simulink model "firebreak_microgrid"  (R2026a)
settings: Solver=ode45  StopTime=86400  MaxStep=0.1
settings Model: Creator=bawan  LastModifiedBy=bawan

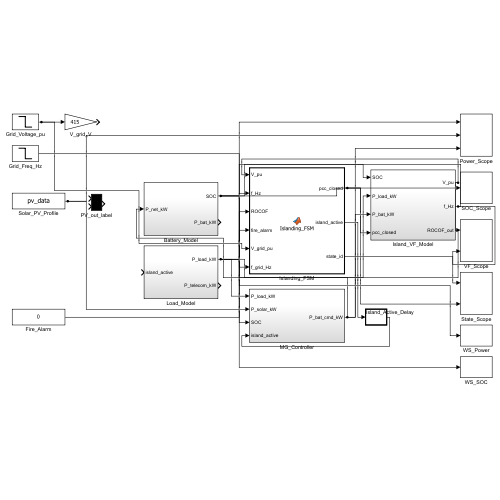
[thumbnail: Simulink's stored preview of the top-level diagram]
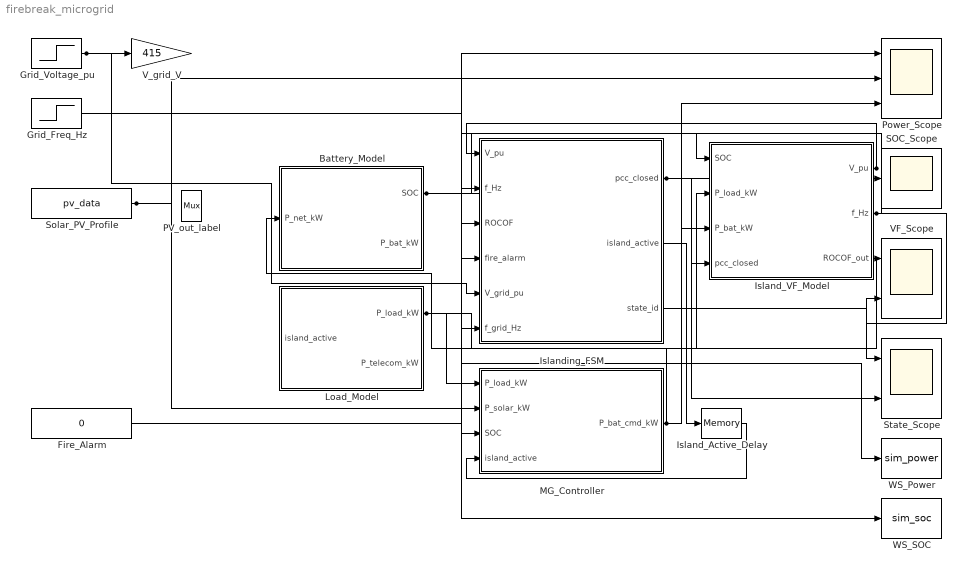
== system firebreak_microgrid ==
  Battery_Model : Subsystem
  Fire_Alarm : Constant  Value=0
  Grid_Freq_Hz : Step  Time=61200  InitialValue=50  FinalValue=0  SampleTime=0
  Grid_Voltage_pu : Step  Time=61200  InitialValue=1.0  FinalValue=0.0  SampleTime=0
  Island_Active_Delay : Memory
  Island_VF_Model : Subsystem
  Islanding_FSM : MATLAB Function  TreatAsAtomicUnit=on
  Load_Model : Subsystem
  MG_Controller : Subsystem
  PV_out_label : Mux  Inputs=2
  Power_Scope : Scope  NumInputPorts=3
  SOC_Scope : Scope
  Solar_PV_Profile : FromWorkspace  VariableName=pv_data  OutputAfterFinalValue=Holding final value
  State_Scope : Scope  NumInputPorts=2
  VF_Scope : Scope  NumInputPorts=2
  V_grid_V : Gain  Gain=415
  WS_Power : ToWorkspace  VariableName=sim_power  SaveFormat=Timeseries  SampleTime=-1
  WS_SOC : ToWorkspace  VariableName=sim_soc  SaveFormat=Timeseries  SampleTime=-1
  wires:
  Grid_Voltage_pu/1 -> V_grid_V/1, Islanding_FSM/5(V_grid_pu)
  Solar_PV_Profile/1 -> MG_Controller/2(P_solar_kW), Power_Scope/2
  Load_Model/1(P_load_kW) -> MG_Controller/1(P_load_kW), Island_VF_Model/2(P_load_kW), Power_Scope/1, WS_Power/1
  Battery_Model/1(SOC) -> MG_Controller/3(SOC), Island_VF_Model/1(SOC), SOC_Scope/1, WS_SOC/1
  Islanding_FSM/2(island_active) -> Island_Active_Delay/1
  Island_Active_Delay/1 -> MG_Controller/4(island_active)
  MG_Controller/1(P_bat_cmd_kW) -> Island_VF_Model/3(P_bat_kW), Battery_Model/1(P_net_kW), Power_Scope/3
  Islanding_FSM/1(pcc_closed) -> Island_VF_Model/4(pcc_closed), State_Scope/2
  Fire_Alarm/1 -> Islanding_FSM/4(fire_alarm)
  Grid_Freq_Hz/1 -> Islanding_FSM/6(f_grid_Hz)
  Island_VF_Model/1(V_pu) -> Islanding_FSM/1(V_pu), VF_Scope/1
  Island_VF_Model/2(f_Hz) -> Islanding_FSM/2(f_Hz), VF_Scope/2
  Island_VF_Model/3(ROCOF_out) -> Islanding_FSM/3(ROCOF)
  Islanding_FSM/3(state_id) -> State_Scope/1

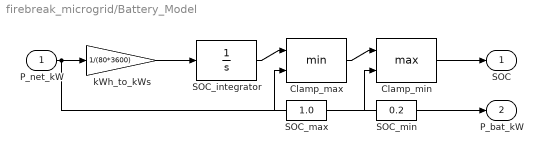
== system firebreak_microgrid/Battery_Model ==
  P_net_kW : Inport
  Clamp_max : MinMax  Inputs=2
  Clamp_min : MinMax  Function=max  Inputs=2
  SOC_integrator : Integrator  InitialCondition=1
  SOC_max : Constant  Value=1.0
  SOC_min : Constant  Value=0.2
  kWh_to_kWs : Gain  Gain=1/(80*3600)
  SOC : Outport
  P_bat_kW : Outport  Port=2
  wires:
  P_net_kW/1 -> kWh_to_kWs/1, P_bat_kW/1
  kWh_to_kWs/1 -> SOC_integrator/1
  SOC_integrator/1 -> Clamp_max/1
  SOC_max/1 -> Clamp_max/2
  Clamp_max/1 -> Clamp_min/1
  SOC_min/1 -> Clamp_min/2
  Clamp_min/1 -> SOC/1

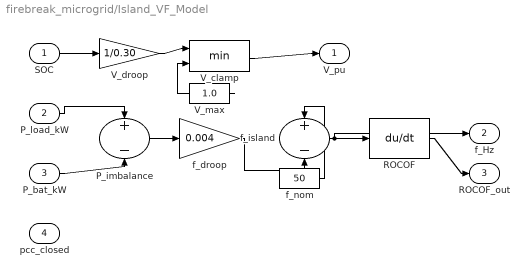
== system firebreak_microgrid/Island_VF_Model ==
  SOC : Inport
  P_load_kW : Inport  Port=2
  P_bat_kW : Inport  Port=3
  pcc_closed : Inport  Port=4
  P_imbalance : Sum  Inputs=+-
  ROCOF : Derivative
  V_clamp : MinMax  Inputs=2
  V_droop : Gain  Gain=1/0.30
  V_max : Constant  Value=1.0
  f_droop : Gain  Gain=0.004
  f_island : Sum  Inputs=+-
  f_nom : Constant  Value=50
  V_pu : Outport
  f_Hz : Outport  Port=2
  ROCOF_out : Outport  Port=3
  wires:
  SOC/1 -> V_droop/1
  V_droop/1 -> V_clamp/1
  V_max/1 -> V_clamp/2
  P_load_kW/1 -> P_imbalance/1
  P_bat_kW/1 -> P_imbalance/2
  P_imbalance/1 -> f_droop/1
  f_nom/1 -> f_island/1
  f_droop/1 -> f_island/2
  f_island/1 -> ROCOF/1, f_Hz/1
  V_clamp/1 -> V_pu/1
  ROCOF/1 -> ROCOF_out/1

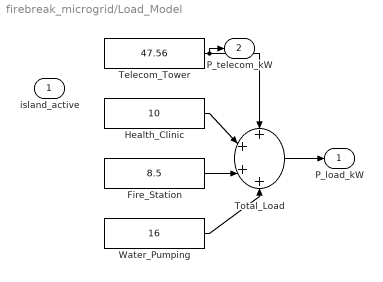
== system firebreak_microgrid/Load_Model ==
  island_active : Inport
  Fire_Station : Constant  Value=8.5
  Health_Clinic : Constant  Value=10
  Telecom_Tower : Constant  Value=47.56
  Total_Load : Sum  Inputs=++++
  Water_Pumping : Constant  Value=16
  P_load_kW : Outport
  P_telecom_kW : Outport  Port=2
  wires:
  Telecom_Tower/1 -> Total_Load/1, P_telecom_kW/1
  Health_Clinic/1 -> Total_Load/2
  Fire_Station/1 -> Total_Load/3
  Water_Pumping/1 -> Total_Load/4
  Total_Load/1 -> P_load_kW/1

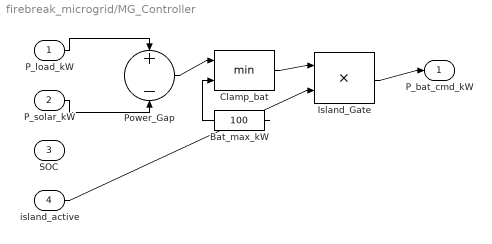
== system firebreak_microgrid/MG_Controller ==
  P_load_kW : Inport
  P_solar_kW : Inport  Port=2
  SOC : Inport  Port=3
  island_active : Inport  Port=4
  Bat_max_kW : Constant  Value=100
  Clamp_bat : MinMax  Inputs=2
  Island_Gate : Product
  Power_Gap : Sum  Inputs=+-
  P_bat_cmd_kW : Outport
  wires:
  P_load_kW/1 -> Power_Gap/1
  P_solar_kW/1 -> Power_Gap/2
  Power_Gap/1 -> Clamp_bat/1
  Bat_max_kW/1 -> Clamp_bat/2
  Clamp_bat/1 -> Island_Gate/1
  island_active/1 -> Island_Gate/2
  Island_Gate/1 -> P_bat_cmd_kW/1

== matlab function firebreak_microgrid/Islanding_FSM ==
  data: V_pu input; pcc_closed output; f_Hz input; ROCOF input; fire_alarm input; V_grid_pu input; f_grid_Hz input; island_active output; state_id output
function [pcc_closed, island_active, state_id] = Islanding_FSM(...
    V_pu, f_Hz, ROCOF, fire_alarm, V_grid_pu, f_grid_Hz)
%#codegen
% Islanding state machine for Firebreak Microgrid
% AS/NZS 4777.2 compliant loss-of-supply detection
%
% States:
%   0 = GRID_CONNECTED  — normal, PCC closed
%   1 = ISLANDED        — PCC open, battery supplies load
%   2 = RESYNC_CHECK    — grid back, checking conditions
%   3 = RECONNECTED     — PCC reclosed, back to grid

% Thresholds (AS/NZS 4777.2)
UV_thresh   = 0.85;   % Under-voltage (pu)
OV_thresh   = 1.10;   % Over-voltage (pu)
UF_thresh   = 49.0;   % Under-frequency (Hz)
OF_thresh   = 51.0;   % Over-frequency (Hz)
ROCOF_thresh= 1.0;    % Rate of change of frequency (Hz/s)
resync_dV   = 0.05;   % Resync ΔV tolerance (pu)
resync_df   = 0.10;   % Resync Δf tolerance (Hz)

% Persistent state
persistent state;
if isempty(state), state = 0; end

% Default outputs (required by codegen — overwritten below)
pcc_closed    = 1.0;   % PCC closed by default
island_active = 0.0;   % not islanded by default
state_id      = 0.0;   % GRID_CONNECTED by default

% --- Loss of supply detection ---
uv_trip    = (V_pu < UV_thresh) || (V_pu > OV_thresh);
uf_trip    = (f_Hz < UF_thresh) || (f_Hz > OF_thresh);
rocof_trip = (abs(ROCOF) > ROCOF_thresh);
fire_trip  = logical(fire_alarm);
loss_detected = uv_trip || uf_trip || rocof_trip || fire_trip;

% --- Grid returned check ---
grid_ok = (V_grid_pu > 0.95) && (V_grid_pu < 1.05) && ...
          (f_grid_Hz > 49.5) && (f_grid_Hz < 50.5);

% --- Resync conditions (AS/NZS 4777.2 reconnect) ---
dV = abs(V_pu - V_grid_pu);
df = abs(f_Hz - f_grid_Hz);
resync_ok = grid_ok && (dV < resync_dV) && (df < resync_df) && ~fire_trip;

% --- State transitions ---
switch state
    case 0  % GRID_CONNECTED
        if loss_detected
            state = 1;  % → ISLANDED
        end

    case 1  % ISLANDED
        if grid_ok && ~fire_trip
            state = 2;  % → RESYNC_CHECK
        end

    case 2  % RESYNC_CHECK
        if resync_ok
            state = 3;  % → RECONNECTED
        elseif ~grid_ok || fire_trip
            state = 1;  % Back to ISLANDED
        end

    case 3  % RECONNECTED
        if loss_detected
            state = 1;  % Trip again if needed
        else
            state = 0;  % Back to normal
        end
end

% --- Outputs ---
pcc_closed    = double(state ~= 1);  % Open only when ISLANDED
island_active = double(state == 1 || state == 2);
state_id      = double(state);
